simulink model "linearized_model"  (R2023a)
settings: Solver=ode23t  StartTime=0.0  StopTime=100  RelTol=1e-3
values from neighbouring files (symbols this model uses):
  A = [0 0 0 1 0 0 ... (first row only)    [nl_parameters_3D.m]
  B = [0 0 ... (first row only)    [nl_parameters_3D.m]
  eps0 = 0    [nl_parameters_3D.m]
  eps0dot = 0    [nl_parameters_3D.m]
  lam0 = 0    [nl_parameters_3D.m]
  lam0dot = 0    [nl_parameters_3D.m]
  p1 = (-(Mf+Mb)*g*La+Mc*g*Lc)/Jeps    (= -1.5604744186)    [nl_parameters_3D.m]
  p10 = -Km*La/Jlam    (= -0.0907317073171)    [nl_parameters_3D.m]
  p2 = (-(Mf+Mb)*g*(Ld+Le)+Mc*g*Ld)/Jeps    (= -0.169963953488)    [nl_parameters_3D.m]
  p3 = -Neps/Jeps    (= -0.00116279069767)    [nl_parameters_3D.m]
  p4 = Km*La/Jeps    (= 0.086511627907)    [nl_parameters_3D.m]
  p5 = (-Mf+Mb)*g*Lh/Jro    (= 0)    [nl_parameters_3D.m]
  p6 = -(Mf+Mb)*g*Le/Jro    (= -6.33190909091)    [nl_parameters_3D.m]
  p7 = -Nro/Jro    (= -0.0227272727273)    [nl_parameters_3D.m]
  p8 = Km*Lh/Jro    (= 0.490909090909)    [nl_parameters_3D.m]
  p9 = -Nlam/Jlam    (= -0.00609756097561)    [nl_parameters_3D.m]
  ro0 = 0    [nl_parameters_3D.m]
  ro0dot = 0    [nl_parameters_3D.m]
  u0 = [Vf0;Vb0]    [nl_parameters_3D.m]
  Vb0 = double(Vb0)    [nl_parameters_3D.m]
  Vf0 = double(Vf0)    [nl_parameters_3D.m]
  x0 = [eps0; ro0; lam0; eps0dot; ro0dot; lam0dot]    [nl_parameters_3D.m]
settings Model: Creator=Diego Jauregui  LastModifiedBy=meng_fanze
settings SolverCC: AlgebraicLoopSolver=TrustRegion
settings DataIOCC: ReturnWorkspaceOutputs=off
settings DebuggingCC: UnconnectedInputMsg=warning  UnconnectedOutputMsg=warning  UnconnectedLineMsg=warning  ArithmeticOperatorsInVariantConditions=warning
settings ModelReferenceCC: EnableRefExpFcnMdlSchedulingChecks=on
settings SFSimCC: SimUseLocalCustomCode=off  CustomCodeUndefinedFunction=UseInterfaceOnly
settings RTWCC: RTWUseLocalCustomCode=off

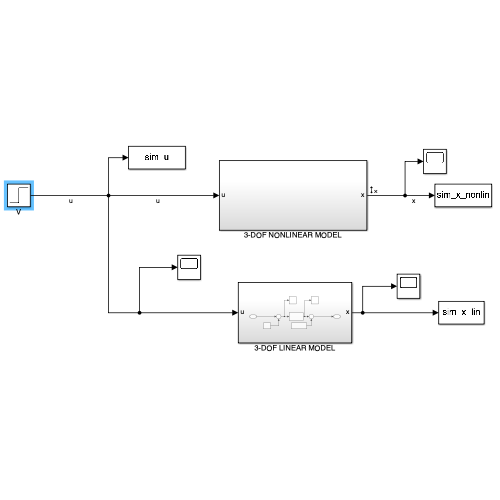
[thumbnail: Simulink's stored preview of the top-level diagram]
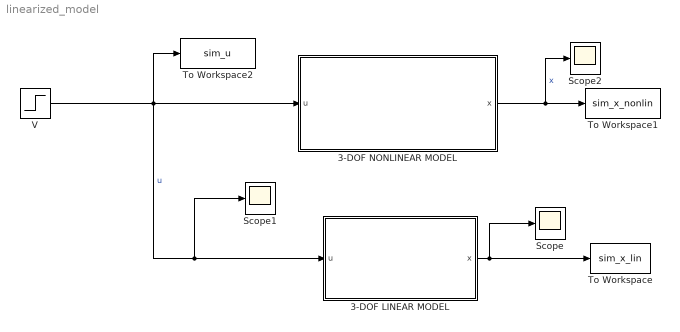
== system linearized_model ==
  3-DOF LINEAR MODEL : Subsystem
  3-DOF NONLINEAR MODEL : Subsystem
  Scope : Scope
  Scope1 : Scope
  Scope2 : Scope
  To Workspace : ToWorkspace  VariableName=sim_x_lin  SaveFormat=Timeseries  SampleTime=-1
  To Workspace1 : ToWorkspace  VariableName=sim_x_nonlin  SaveFormat=Timeseries  SampleTime=-1
  To Workspace2 : ToWorkspace  VariableName=sim_u  SaveFormat=Timeseries  SampleTime=-1
  V : Step  Time=0  After=[Vf0;Vb0]  SampleTime=0
  wires:
  V/1 -> 3-DOF NONLINEAR MODEL/1(u), To Workspace2/1, Scope1/1, 3-DOF LINEAR MODEL/1(u)  "u"
  3-DOF NONLINEAR MODEL/1(x) -> Scope2/1, To Workspace1/1  "x"
  3-DOF LINEAR MODEL/1(x) -> To Workspace/1, Scope/1

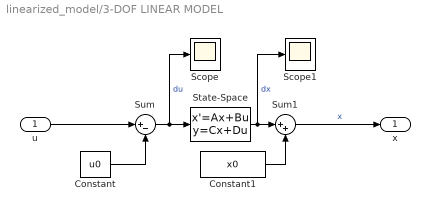
== system linearized_model/3-DOF LINEAR MODEL ==
  u : Inport
  Constant : Constant  Value=u0
  Constant1 : Constant  Value=x0
  Scope : Scope
  Scope1 : Scope
  State-Space : StateSpace  A=A  B=B  C=eye(size(A))  D=zeros(size(B))  InitialCondition=x0  ContinuousStateAttributes={'eps','ro','lam','epsdot','rodot','lamdot'}
  Sum : Sum  Inputs=|+-
  Sum1 : Sum  Inputs=|++
  x : Outport  VectorParamsAs1DForOutWhenUnconnected=off
  wires:
  State-Space/1 -> Scope1/1, Sum1/1  "dx"
  Sum1/1 -> x/1  "x"
  Sum/1 -> Scope/1, State-Space/1  "du"
  Constant1/1 -> Sum1/2
  u/1 -> Sum/1
  Constant/1 -> Sum/2

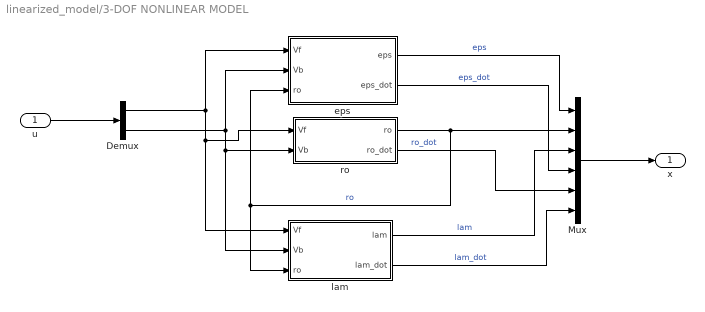
== system linearized_model/3-DOF NONLINEAR MODEL ==
  u : Inport
  Demux : Demux  Outputs=2
  Mux : Mux  Inputs=6
  eps : Subsystem
  lam : Subsystem
  ro : Subsystem
  x : Outport  VectorParamsAs1DForOutWhenUnconnected=off
  wires:
  u/1 -> Demux/1
  Demux/1 -> eps/1(Vf), ro/1(Vf), lam/1(Vf)
  Demux/2 -> eps/2(Vb), lam/2(Vb), ro/2(Vb)
  ro/1(ro) -> Mux/2, eps/3(ro), lam/3(ro)  "ro"
  Mux/1 -> x/1
  eps/1(eps) -> Mux/1  "eps"
  lam/1(lam) -> Mux/3  "lam"
  eps/2(eps_dot) -> Mux/4  "eps_dot"
  ro/2(ro_dot) -> Mux/5  "ro_dot"
  lam/2(lam_dot) -> Mux/6  "lam_dot"

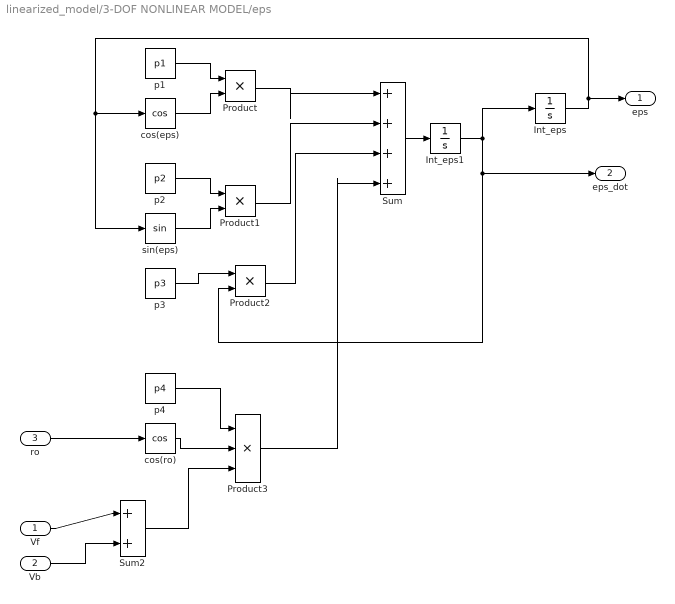
== system linearized_model/3-DOF NONLINEAR MODEL/eps ==
  Vf : Inport
  Vb : Inport  Port=2
  ro : Inport  Port=3
  Int_eps : Integrator  InitialCondition=eps0  ContinuousStateAttributes='eps'
  Int_eps1 : Integrator  InitialCondition=eps0dot  ContinuousStateAttributes='epsdot'
  Product : Product  RndMeth=Zero
  Product1 : Product  RndMeth=Zero
  Product2 : Product  RndMeth=Zero
  Product3 : Product  Inputs=3  RndMeth=Zero
  Sum : Sum  Inputs=|++++
  Sum2 : Sum  Inputs=|++
  cos(eps) : Trigonometry  Operator=cos
  cos(ro) : Trigonometry  Operator=cos
  p1 : Constant  Value=p1
  p2 : Constant  Value=p2
  p3 : Constant  Value=p3
  p4 : Constant  Value=p4
  sin(eps) : Trigonometry
  eps : Outport  VectorParamsAs1DForOutWhenUnconnected=off
  eps_dot : Outport  Port=2  VectorParamsAs1DForOutWhenUnconnected=off
  wires:
  Int_eps/1 -> cos(eps)/1, sin(eps)/1, eps/1
  p1/1 -> Product/1
  cos(eps)/1 -> Product/2
  Product/1 -> Sum/1
  p2/1 -> Product1/1
  sin(eps)/1 -> Product1/2
  Product1/1 -> Sum/2
  p3/1 -> Product2/1
  Product2/1 -> Sum/3
  p4/1 -> Product3/1
  cos(ro)/1 -> Product3/2
  ro/1 -> cos(ro)/1
  Product3/1 -> Sum/4
  Sum/1 -> Int_eps1/1
  Int_eps1/1 -> Product2/2, eps_dot/1, Int_eps/1
  Vf/1 -> Sum2/1
  Vb/1 -> Sum2/2
  Sum2/1 -> Product3/3

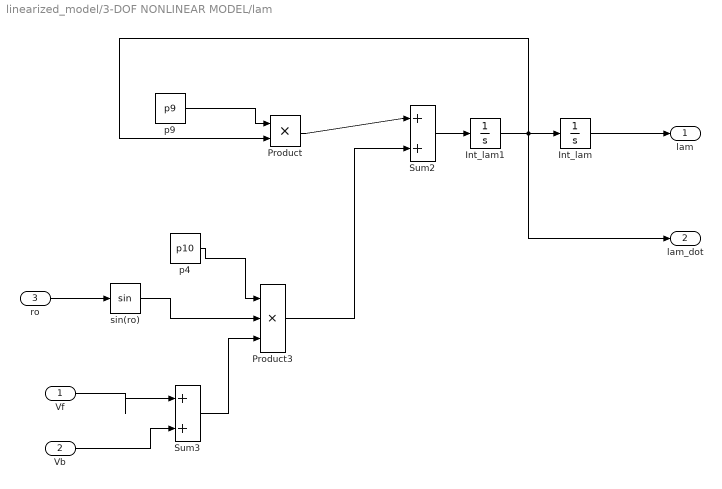
== system linearized_model/3-DOF NONLINEAR MODEL/lam ==
  Vf : Inport
  Vb : Inport  Port=2
  ro : Inport  Port=3
  Int_lam : Integrator  InitialCondition=lam0  ContinuousStateAttributes='lam'
  Int_lam1 : Integrator  InitialCondition=lam0dot  ContinuousStateAttributes='lamdot'
  Product : Product  RndMeth=Zero
  Product3 : Product  Inputs=3  RndMeth=Zero
  Sum2 : Sum  Inputs=|++
  Sum3 : Sum  Inputs=|++
  p4 : Constant  Value=p10
  p9 : Constant  Value=p9
  sin(ro) : Trigonometry
  lam : Outport  VectorParamsAs1DForOutWhenUnconnected=off
  lam_dot : Outport  Port=2  VectorParamsAs1DForOutWhenUnconnected=off
  wires:
  Int_lam/1 -> lam/1
  p9/1 -> Product/1
  p4/1 -> Product3/1
  sin(ro)/1 -> Product3/2
  ro/1 -> sin(ro)/1
  Product/1 -> Sum2/1
  Sum2/1 -> Int_lam1/1
  Product3/1 -> Sum2/2
  Int_lam1/1 -> lam_dot/1, Product/2, Int_lam/1
  Vf/1 -> Sum3/1
  Vb/1 -> Sum3/2
  Sum3/1 -> Product3/3

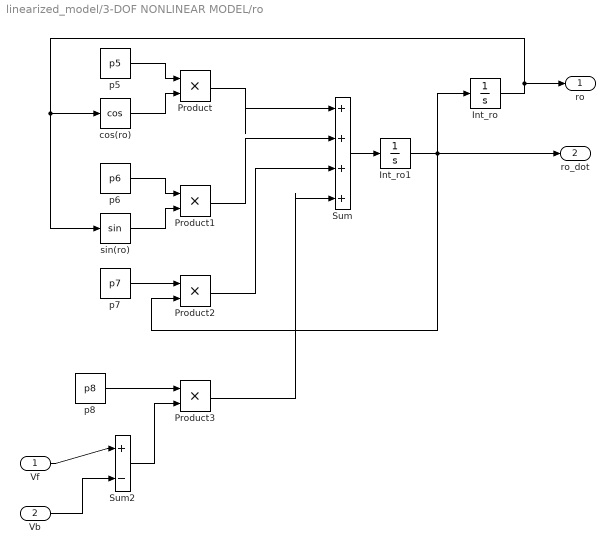
== system linearized_model/3-DOF NONLINEAR MODEL/ro ==
  Vf : Inport
  Vb : Inport  Port=2
  Int_ro : Integrator  InitialCondition=ro0  ContinuousStateAttributes='ro'
  Int_ro1 : Integrator  InitialCondition=ro0dot  ContinuousStateAttributes='rodot'
  Product{,1..3} (4 alike) : Product  RndMeth=Zero
  Sum : Sum  Inputs=|++++
  Sum2 : Sum  Inputs=|+-
  cos(ro) : Trigonometry  Operator=cos
  p5 : Constant  Value=p5
  p6 : Constant  Value=p6
  p7 : Constant  Value=p7
  p8 : Constant  Value=p8
  sin(ro) : Trigonometry
  ro : Outport  VectorParamsAs1DForOutWhenUnconnected=off
  ro_dot : Outport  Port=2  VectorParamsAs1DForOutWhenUnconnected=off
  wires:
  Int_ro/1 -> cos(ro)/1, sin(ro)/1, ro/1
  p5/1 -> Product/1
  cos(ro)/1 -> Product/2
  Product/1 -> Sum/1
  p6/1 -> Product1/1
  sin(ro)/1 -> Product1/2
  Product1/1 -> Sum/2
  p7/1 -> Product2/1
  Product2/1 -> Sum/3
  p8/1 -> Product3/1
  Product3/1 -> Sum/4
  Int_ro1/1 -> Product2/2, ro_dot/1, Int_ro/1
  Sum/1 -> Int_ro1/1
  Vf/1 -> Sum2/1
  Vb/1 -> Sum2/2
  Sum2/1 -> Product3/2
